simulink model "FinalLongitudinalDynamics"  (R2014a)
settings: Solver=ode45  StartTime=0.0  StopTime=50  RelTol=1e-3
values from neighbouring files (symbols this model uses):
  a_theta1 = -rho*Va^2*c*S/(2*Jy)*Cm_q*c/(2*Va)    (= -14.426787663)    [MAINLongitudinal.m]
  a_theta2 = -rho*Va^2*c*S*Cm_alpha/(2*Jy)    (= 147.205731874)    [MAINLongitudinal.m]
  a_theta3 = rho*Va^2*c*S*Cm_deltaE/(2*Jy)    (= -165.053071401)    [MAINLongitudinal.m]
  kd_theta = (2*zeta_theta*w_ntheta-a_theta1)/a_theta3    [MAINLongitudinal.m]
  kI_h = 2*zeta_h*wn_h/(K_thetaDC*Va)    [MAINLongitudinal.m]
  kp_h = wn_h^2/(K_thetaDC*Va)    [MAINLongitudinal.m]
  kp_theta = deltaElevator_max/e_thetamax*sign(a_theta3)    [MAINLongitudinal.m]
  Va = 10    [MAIN.m]    (also in MAINLongitudinal.m)
settings Model: Creator=Nathan  LastModifiedBy=Nathan

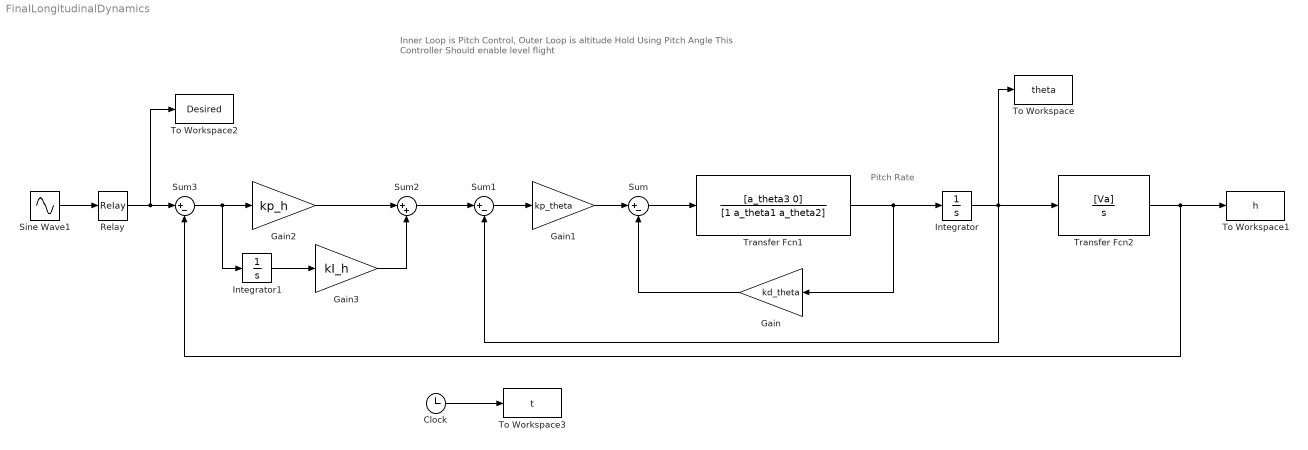
== system FinalLongitudinalDynamics ==
  note: Inner Loop is Pitch Control, Outer Loop is altitude Hold Using Pitch Angle
      | This Controller Should enable level flight
  note: Pitch Rate
  Clock : Clock
  Gain : Gain  Gain=kd_theta
  Gain1 : Gain  Gain=kp_theta
  Gain2 : Gain  Gain=kp_h
  Gain3 : Gain  Gain=kI_h
  Integrator : Integrator
  Integrator1 : Integrator
  Relay : Relay  OnOutputValue=10  OffOutputValue=-10
  Sine Wave1 : Sin  Amplitude=40  Frequency=.1  SampleTime=0
  Sum : Sum  Inputs=|+-
  Sum1 : Sum  Inputs=|+-
  Sum2 : Sum  Inputs=|++
  Sum3 : Sum  Inputs=|+-
  To Workspace : ToWorkspace  VariableName=theta  SampleTime=-1
  To Workspace1 : ToWorkspace  VariableName=h  SampleTime=-1
  To Workspace2 : ToWorkspace  VariableName=Desired  SampleTime=-1
  To Workspace3 : ToWorkspace  VariableName=t  SampleTime=-1
  Transfer Fcn1 : TransferFcn  Numerator=[a_theta3 0]  Denominator=[1 a_theta1 a_theta2]
  Transfer Fcn2 : TransferFcn  Numerator=[Va]  Denominator=[1 0]
  wires:
  Transfer Fcn1/1 -> Integrator/1, Gain/1
  Gain/1 -> Sum/2
  Gain1/1 -> Sum/1
  Sum/1 -> Transfer Fcn1/1
  Integrator/1 -> Transfer Fcn2/1, To Workspace/1, Sum1/2
  Sum1/1 -> Gain1/1
  Sine Wave1/1 -> Relay/1
  Clock/1 -> To Workspace3/1
  Transfer Fcn2/1 -> Sum3/2, To Workspace1/1
  Sum2/1 -> Sum1/1
  Gain3/1 -> Sum2/2
  Gain2/1 -> Sum2/1
  Sum3/1 -> Integrator1/1, Gain2/1
  Integrator1/1 -> Gain3/1
  Relay/1 -> To Workspace2/1, Sum3/1
